simulink model "mc64_hb_43_newquant"  (Simulink 7.6)
settings: Solver=ode45  StartTime=0.0  StopTime=5000  RelTol=1e-3
libraries: xbsIndex_r4 x1281, xps_library x27, casper_library_misc x17, dspsigops x8
(part 1 of 13)
settings Model: Creator=hong  LastModifiedBy=hong

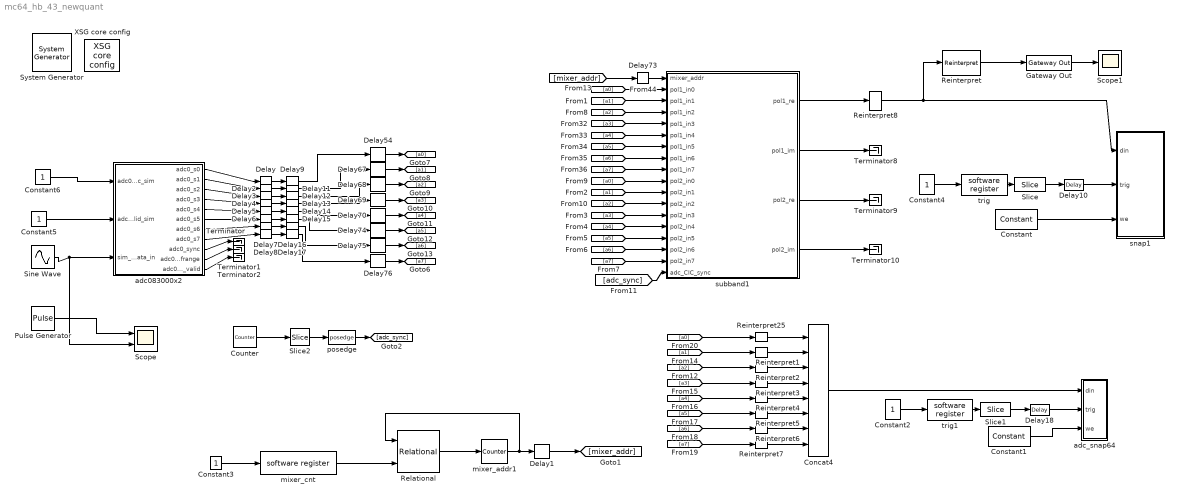
== system mc64_hb_43_newquant ==
  " System Generator" : xbsIndex_r4/ System Generator  Tag=genX  SystemSampleTime=-1  xilinxfamily=virtex5  part=xc5vsx95t  speed=-1  package=ff1136  synthesis_tool=XST  clock_wrapper=Clock Enables  directory=./mc64_hb_43_noise/sysgen  proj_type=Project Navigator  Synth_file=XST Defaults  Impl_file=ISE Defaults  testbench=off  simulink_period=1  sysclk_period=6.6667  dcm_input_clock_period=100  incr_netlist=off  trim_vbits=Everywhere in SubSystem  dbl_ovrd=According to Block Masks  core_generation=According to Block Masks  run_coregen=off  deprecated_control=off  eval_field=0  block_type=sysgen
  Concat4 : xbsIndex_r4/Concat  num_inputs=8  dbl_ovrd=off  block_type=concat
  Constant : xbsIndex_r4/Constant  const=1  gui_display_data_type=Boolean  arith_type=Boolean  n_bits=16  bin_pt=14  preci_type=Single  exp_width=8  frac_width=24  explicit_period=off  period=1  equ=P=C  opselect=C  inp2=PCIN>>17  opr=+  inp1=P  carry=CIN  dbl_ovrd=off  block_type=constant
  Constant1 : xbsIndex_r4/Constant  const=1  gui_display_data_type=Boolean  arith_type=Boolean  n_bits=16  bin_pt=14  preci_type=Single  exp_width=8  frac_width=24  explicit_period=off  period=1  equ=P=C  opselect=C  inp2=PCIN>>17  opr=+  inp1=P  carry=CIN  dbl_ovrd=off  block_type=constant
  Constant{2..6} (5 alike) : Constant
  Counter : xbsIndex_r4/Counter  cnt_type=Free Running  cnt_to=Inf  operation=Up  start_count=0  cnt_by_val=1  arith_type=Unsigned  n_bits=16  bin_pt=0  load_pin=off  rst=off  en=off  explicit_period=on  period=1  dbl_ovrd=off  use_behavioral_HDL=off  implementation=Fabric  block_type=counter
  Delay{,2..8} (8 alike) : xbsIndex_r4/Delay  rst=off  infoeditControl=Selection of Reset will increase slice count due to use of real FFs and instead of SRLs  en=off  latency=3  dbl_ovrd=off  reg_retiming=off  block_type=delay
  Delay1 : xbsIndex_r4/Delay  rst=off  infoeditControl=Selection of Reset will increase slice count due to use of real FFs and instead of SRLs  en=off  latency=2  dbl_ovrd=off  reg_retiming=on  block_type=delay
      settings: block_version=11.4
  Delay10 : xbsIndex_r4/Delay  rst=off  infoeditControl=Selection of Reset will increase slice count due to use of real FFs and instead of SRLs  en=off  latency=20  dbl_ovrd=off  reg_retiming=off  block_type=delay
  Delay{9,11..17} (8 alike) : xbsIndex_r4/Delay  rst=off  infoeditControl=Selection of Reset will increase slice count due to use of real FFs and instead of SRLs  en=off  latency=8  dbl_ovrd=off  reg_retiming=off  block_type=delay
  Delay18 : xbsIndex_r4/Delay  rst=off  infoeditControl=Selection of Reset will increase slice count due to use of real FFs and instead of SRLs  en=off  latency=20  dbl_ovrd=off  reg_retiming=off  block_type=delay
  Delay{54,67..70,74..76} (8 alike) : xbsIndex_r4/Delay  rst=off  infoeditControl=Selection of Reset will increase slice count due to use of real FFs and instead of SRLs  en=off  latency=3  dbl_ovrd=off  reg_retiming=on  block_type=delay
      settings: block_version=11.4
  Delay73 : xbsIndex_r4/Delay  rst=off  infoeditControl=Selection of Reset will increase slice count due to use of real FFs and instead of SRLs  en=off  latency=5  dbl_ovrd=off  reg_retiming=on  block_type=delay
      settings: block_version=11.4
  Gateway Out : xbsIndex_r4/Gateway Out  hdl_port=on  timing_constraint=None  locs_specified=off  LOCs={}  block_type=gatewayout
      settings: infoedit="Gateway out block.  Converts Xilinx fixed point or floating-point type inputs into ouputs of type Simulink integer, double, or fixed point.<br><br>Hardware notes:  In hardware these blocks become top level output ports or are discarded, depending on how they are configured."
  Pulse Generator : DiscretePulseGenerator  Period=480
  Reinterpret : xbsIndex_r4/Reinterpret  force_arith_type=on  arith_type="Signed  (2's comp)"  force_bin_pt=on  bin_pt=31  block_type=reinterpret
  Reinterpret{1..8,25} (9 alike) : xbsIndex_r4/Reinterpret  force_arith_type=on  arith_type=Unsigned  force_bin_pt=on  bin_pt=0  block_type=reinterpret
  Relational : xbsIndex_r4/Relational  mode=a=b  en=off  latency=1  dbl_ovrd=off  block_type=relational
  Scope : Scope  NumInputPorts=2
      settings: YMin=-5~-5  YMax=5~5
  Scope1 : Scope
      settings: TimeRange=746.6442953020135  YMin=-4e-05  YMax=4e-05  SaveName=ScopeData2
  Sine Wave : Sin  Frequency=(pi/2)*(2^1)-(pi/2)*(2^-1)  Samples=200  SampleTime=1/8
  Slice : xbsIndex_r4/Slice  nbits=1  boolean_output=on  mode=Lower Bit Location + Width  bit1=0  base1=MSB of Input  bit0=0  base0=LSB of Input  dbl_ovrd=off  block_type=slice
  Slice1 : xbsIndex_r4/Slice  nbits=1  boolean_output=on  mode=Lower Bit Location + Width  bit1=0  base1=MSB of Input  bit0=0  base0=LSB of Input  dbl_ovrd=off  block_type=slice
  Slice2 : xbsIndex_r4/Slice  nbits=1  boolean_output=on  mode=Upper Bit Location + Width  bit1=0  base1=MSB of Input  bit0=0  base0=LSB of Input  dbl_ovrd=off  block_type=slice
  Terminator{,1..2,8..10} (6 alike) : Terminator
  XSG core config : xps_library/XSG core config  Tag=xps:xsg  SystemSampleTime=-1  hw_sys=ROACH:sx95t  ibob_linux=off  clk_src=adc0_clk  iBOB_clk_src=sys_clk  BEE2_ctrl_clk_src=sys_clk  BEE2_usr_clk_src=sys_clk  ROACH_clk_src=adc0_clk  ROACH2_clk_src=adc0_clk  CORR_clk_src=sys_clk  gpio_clk_io_group=iBOB:sma  gpio_clk_bit_index=0  clk_rate=150  sample_period=1  synthesis_tool=XST  mpc_type=powerpc440_ext
  adc083000x2 : Subsystem  Tag=xps:adc083000x2  AncestorBlock=xps_library/adc083000x2  mask(adc_083000x2){use_adc0=on, use_adc1=off, demux_adc=off, clock_sync=off, verbose=off, using_ctrl=on, adc_clk_rate=800, sample_period=1, bit_width=8}
      mask prompts: use_adc0 "Use ZD0K0?"; use_adc1 "Use ZDOK1?"; demux_adc "Demux ADCs by 2?"; clock_sync "Interleave 2 ADC boards?"; verbose "Verbose Block Creation?"; using_ctrl "Add ports for control registers?"; adc_clk_rate "ADC clock rate (MHz)"; sample_period "Sample Period"; bit_width "Output Bit Width"
      mask help:
      | The ADC block converts analog inputs to digital outputs.
      | Every clock cycle, the inputs are sampled and digitized to
      | 8 bit binary point numbers in the range of [-1, 1).
      |
      | Online block-specific documentation: http://casper.berkeley.edu/wiki/Adc083000
      mask init:
      | adc083000_mask;
      mask Help: eval('xlWeb([getenv(''MLIB_ROOT''), ''\doc\html\sys_adc\sys_adc.html''])')
  adc_snap64 : Subsystem  AncestorBlock=casper_library_scopes/snap64  mask(snap64){nsamples=13}
      mask prompts: nsamples "No. of samples(2^?)"
      mask help:
      | The <i>snap</i> block provides a packaged solution to capturing data from
      | the FPGA fabric and making it accessible from the CPU.  The block comes in
      | 2 flavors: <i>snap</i> (which captures to a 32 bit wide Shared BRAM), and
      | <i>snap64</i> (which captures to 2x32 bit wide Shared BRAMs to effect a
      | 64 bit capture).
      mask Help: eval('xlWeb(''http://casper.berkeley.edu/wiki/Snap'')')
  mixer_addr1 : xbsIndex_r4/Counter  cnt_type=Free Running  cnt_to=Inf  operation=Up  start_count=0  cnt_by_val=1  arith_type=Unsigned  n_bits=11  bin_pt=0  load_pin=off  rst=on  en=off  explicit_period=on  period=1  dbl_ovrd=off  use_behavioral_HDL=off  implementation=Fabric  block_type=counter
      settings: block_version=11.4
  mixer_cnt : xps_library/software register  Tag=xps:sw_reg  SystemSampleTime=-1  io_dir=From Processor  arith_type=Unsigned  bitwidth=32  bin_pt=0  sample_period=1  gw_name=mc64_hb_43_noise_mixer_cnt_user_data_out
  posedge : casper_library_misc/posedge  Tag=Rising Edge Detector  SystemSampleTime=-1
  snap1 : Subsystem  AncestorBlock=casper_library_scopes/snap  mask(snap){nsamples=13}
      mask prompts: nsamples "No. of samples(2^?)"
      mask help:
      | The <i>snap</i> block provides a packaged solution to capturing data from
      | the FPGA fabric and making it accessible from the CPU.  The block comes in
      | 2 flavors: <i>snap</i> (which captures to a 32 bit wide Shared BRAM), and
      | <i>snap64</i> (which captures to 2x32 bit wide Shared BRAMs to effect a
      | 64 bit capture).
      mask Help: eval('xlWeb(''http://casper.berkeley.edu/wiki/Snap'')')
  subband1 : Subsystem  mask{mult_latency=5, add_latency=2, bram_length=10}
      mask prompts: mult_latency "Multiplier Latency"; add_latency "Adder Latency"; bram_length "BRAM Length(2^n)"
  trig : xps_library/software register  Tag=xps:sw_reg  SystemSampleTime=-1  io_dir=From Processor  arith_type=Unsigned  bitwidth=32  bin_pt=0  sample_period=1  gw_name=mc64_hb_43_noise_trig_user_data_out
      link override cic_filter_testing_to_compile_trig_user_data_out: arith_type=Unsigned  n_bits=32  bin_pt=0  period=1
  trig1 : xps_library/software register  Tag=xps:sw_reg  SystemSampleTime=-1  io_dir=From Processor  arith_type=Unsigned  bitwidth=32  bin_pt=0  sample_period=1  gw_name=mc64_hb_43_noise_trig1_user_data_out
      link override cic_filter_testing_to_compile_trig_user_data_out: arith_type=Unsigned  n_bits=32  bin_pt=0  period=1
  wires:
  mixer_addr1/1 -> Delay1/1, Relational/1
  Delay1/1 -> [mixer_addr]
  Relational/1 -> mixer_addr1/1
  mixer_cnt/1 -> Relational/2
  Constant3/1 -> mixer_cnt/1
  [mixer_addr] -> Delay73/1
  [a0] -> subband1/2(pol1_in0)
  [a1] -> subband1/3(pol1_in1)
  [a2] -> subband1/4(pol1_in2)
  [a3] -> subband1/5(pol1_in3)
  [a4] -> subband1/6(pol1_in4)
  [a5] -> subband1/7(pol1_in5)
  [a6] -> subband1/8(pol1_in6)
  [a7] -> subband1/9(pol1_in7)
  [a0] -> subband1/10(pol2_in0)
  [a1] -> subband1/11(pol2_in1)
  [a2] -> subband1/12(pol2_in2)
  [a3] -> subband1/13(pol2_in3)
  [a4] -> subband1/14(pol2_in4)
  [a5] -> subband1/15(pol2_in5)
  [a6] -> subband1/16(pol2_in6)
  [a7] -> subband1/17(pol2_in7)
  Delay73/1 -> subband1/1(mixer_addr)
  subband1/1(pol1_re) -> Reinterpret8/1
  [adc_sync] -> subband1/18(adc_CIC_sync)
  Constant/1 -> snap1/3(we)
  Constant4/1 -> trig/1
  trig/1 -> Slice/1
  Slice/1 -> Delay10/1
  Delay10/1 -> snap1/2(trig)
  Concat4/1 -> adc_snap64/1(din)
  Reinterpret25/1 -> Concat4/1
  Reinterpret1/1 -> Concat4/2
  Reinterpret2/1 -> Concat4/3
  Reinterpret3/1 -> Concat4/4
  Reinterpret4/1 -> Concat4/5
  Reinterpret5/1 -> Concat4/6
  Reinterpret6/1 -> Concat4/7
  Reinterpret7/1 -> Concat4/8
  [a0] -> Reinterpret25/1
  [a1] -> Reinterpret1/1
  [a7] -> Reinterpret7/1
  [a6] -> Reinterpret6/1
  [a5] -> Reinterpret5/1
  [a4] -> Reinterpret4/1
  [a3] -> Reinterpret3/1
  [a2] -> Reinterpret2/1
  Constant1/1 -> adc_snap64/3(we)
  Constant2/1 -> trig1/1
  trig1/1 -> Slice1/1
  Slice1/1 -> Delay18/1
  Delay18/1 -> adc_snap64/2(trig)
  Gateway Out/1 -> Scope1/1
  Reinterpret/1 -> Gateway Out/1
  Reinterpret8/1 -> snap1/1(din), Reinterpret/1
  Sine Wave/1 -> Scope/2, adc083000x2/3(sim_adc0_data_in)
  Pulse Generator/1 -> Scope/1
  adc083000x2/1(adc0_s0) -> Delay/1
  adc083000x2/2(adc0_s1) -> Delay2/1
  adc083000x2/3(adc0_s2) -> Delay3/1
  adc083000x2/4(adc0_s3) -> Delay4/1
  adc083000x2/5(adc0_s4) -> Delay5/1
  adc083000x2/6(adc0_s5) -> Delay6/1
  adc083000x2/7(adc0_s6) -> Delay7/1
  adc083000x2/8(adc0_s7) -> Delay8/1
  Delay54/1 -> [a0]
  Delay67/1 -> [a1]
  Delay68/1 -> [a2]
  Delay69/1 -> [a3]
  Delay70/1 -> [a4]
  Delay74/1 -> [a5]
  Delay75/1 -> [a6]
  Delay76/1 -> [a7]
  Delay/1 -> Delay9/1
  Delay2/1 -> Delay11/1
  Delay3/1 -> Delay12/1
  Delay4/1 -> Delay13/1
  Delay5/1 -> Delay14/1
  Delay6/1 -> Delay15/1
  Delay7/1 -> Delay16/1
  Delay8/1 -> Delay17/1
  Delay9/1 -> Delay54/1
  Delay11/1 -> Delay67/1
  Delay12/1 -> Delay68/1
  Delay13/1 -> Delay69/1
  Delay14/1 -> Delay70/1
  Delay15/1 -> Delay74/1
  Delay16/1 -> Delay75/1
  Delay17/1 -> Delay76/1
  Constant5/1 -> adc083000x2/2(adc0_data_valid_sim)
  adc083000x2/9(adc0_sync) -> Terminator/1
  adc083000x2/10(adc0_outofrange) -> Terminator1/1
  adc083000x2/11(adc0_data_valid) -> Terminator2/1
  Counter/1 -> Slice2/1
  Slice2/1 -> posedge/1
  posedge/1 -> [adc_sync]
  Constant6/1 -> adc083000x2/1(adc0_sync_sim)
  subband1/2(pol1_im) -> Terminator8/1
  subband1/3(pol2_re) -> Terminator9/1
  subband1/4(pol2_im) -> Terminator10/1

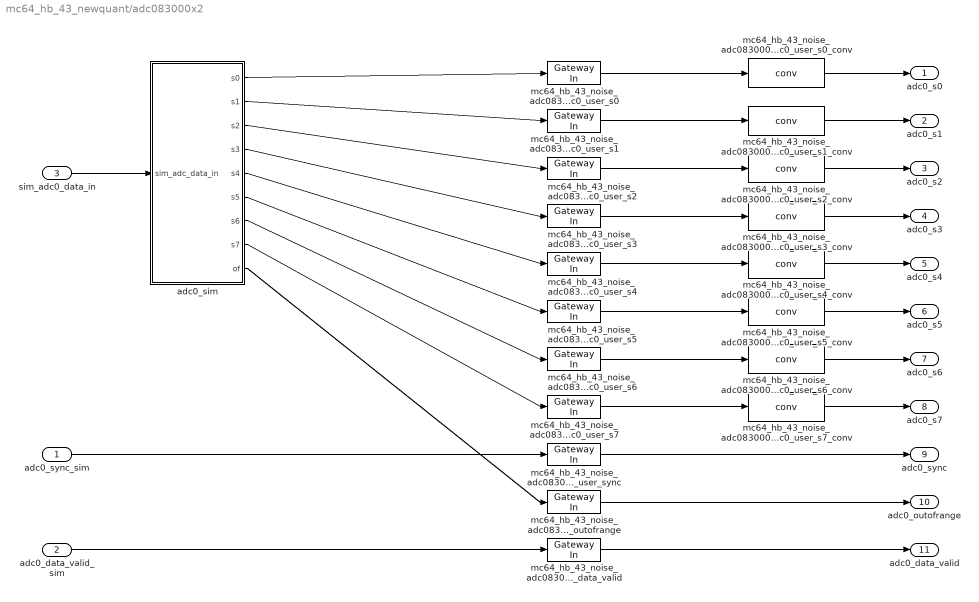
== system mc64_hb_43_newquant/adc083000x2 ==
  adc0_sync_sim : Inport
  adc0_data_valid_sim : Inport  Port=2
  sim_adc0_data_in : Inport  Port=3
  adc0_sim : Subsystem  AncestorBlock=xps_library/ADCs/adc_sim  mask(adc_sim){nStreams=8, bit_width=8}
      mask prompts: nStreams "Number of Output Streams"; bit_width "Sample Bit Width"
      mask help:
      | This block simulates the behavior of a demuxed ADC, which takes
      | as input a waveform and returns digital samples in parallel at
      | a slower rate.
      |
      | This block is used to simulate the behavior
      mask init:
      | adc_sim_init(gcb, ...
      |     'nStreams', nStreams, ...
      |     'bit_width', bit_width);
  mc64_hb_43_noise_adc083000x2_adc0_user_data_valid : xbsIndex_r4/Gateway In  gui_display_data_type=Fixed-point  arith_type=Unsigned  n_bits=1  bin_pt=0  preci_type=Single  exp_width=8  frac_width=24  quantization="Round  (unbiased: +/- Inf)"  overflow=Saturate  period=1  dbl_ovrd=off  timing_constraint=None  locs_specified=off  LOCs={}  hdl_port=on  block_type=gatewayin
      settings: infoedit="Gateway in block.  Converts inputs of type Simulink integer, double and fixed point to  Xilinx fixed point or floating-point data type.<br><br>Hardware notes:  In hardware these blocks become top level input ports."
  mc64_hb_43_noise_adc083000x2_adc0_user_outofrange : xbsIndex_r4/Gateway In  gui_display_data_type=Fixed-point  arith_type=Unsigned  n_bits=4  bin_pt=0  preci_type=Single  exp_width=8  frac_width=24  quantization="Round  (unbiased: +/- Inf)"  overflow=Saturate  period=1  dbl_ovrd=off  timing_constraint=None  locs_specified=off  LOCs={}  hdl_port=on  block_type=gatewayin
      settings: infoedit="Gateway in block.  Converts inputs of type Simulink integer, double and fixed point to  Xilinx fixed point or floating-point data type.<br><br>Hardware notes:  In hardware these blocks become top level input ports."
  mc64_hb_43_noise_adc083000x2_adc0_user_s{0..7} (8 alike) : xbsIndex_r4/Gateway In  gui_display_data_type=Fixed-point  arith_type=Unsigned  n_bits=8  bin_pt=0  preci_type=Single  exp_width=8  frac_width=24  quantization="Round  (unbiased: +/- Inf)"  overflow=Saturate  period=1  dbl_ovrd=off  timing_constraint=None  locs_specified=off  LOCs={}  hdl_port=on  block_type=gatewayin
      settings: infoedit="Gateway in block.  Converts inputs of type Simulink integer, double and fixed point to  Xilinx fixed point or floating-point data type.<br><br>Hardware notes:  In hardware these blocks become top level input ports."
  mc64_hb_43_noise_adc083000x2_adc0_user_s0_conv : xps_library/ADCs/conv  SystemSampleTime=-1  bit_width=8
  mc64_hb_43_noise_adc083000x2_adc0_user_s1_conv : xps_library/ADCs/conv  SystemSampleTime=-1  bit_width=8
  mc64_hb_43_noise_adc083000x2_adc0_user_s2_conv : xps_library/ADCs/conv  SystemSampleTime=-1  bit_width=8
  mc64_hb_43_noise_adc083000x2_adc0_user_s3_conv : xps_library/ADCs/conv  SystemSampleTime=-1  bit_width=8
  mc64_hb_43_noise_adc083000x2_adc0_user_s4_conv : xps_library/ADCs/conv  SystemSampleTime=-1  bit_width=8
  mc64_hb_43_noise_adc083000x2_adc0_user_s5_conv : xps_library/ADCs/conv  SystemSampleTime=-1  bit_width=8
  mc64_hb_43_noise_adc083000x2_adc0_user_s6_conv : xps_library/ADCs/conv  SystemSampleTime=-1  bit_width=8
  mc64_hb_43_noise_adc083000x2_adc0_user_s7_conv : xps_library/ADCs/conv  SystemSampleTime=-1  bit_width=8
  mc64_hb_43_noise_adc083000x2_adc0_user_sync : xbsIndex_r4/Gateway In  gui_display_data_type=Fixed-point  arith_type=Unsigned  n_bits=4  bin_pt=0  preci_type=Single  exp_width=8  frac_width=24  quantization="Round  (unbiased: +/- Inf)"  overflow=Saturate  period=1  dbl_ovrd=off  timing_constraint=None  locs_specified=off  LOCs={}  hdl_port=on  block_type=gatewayin
      settings: infoedit="Gateway in block.  Converts inputs of type Simulink integer, double and fixed point to  Xilinx fixed point or floating-point data type.<br><br>Hardware notes:  In hardware these blocks become top level input ports."
  adc0_s0 : Outport
  adc0_s1 : Outport  Port=2
  adc0_s2 : Outport  Port=3
  adc0_s3 : Outport  Port=4
  adc0_s4 : Outport  Port=5
  adc0_s5 : Outport  Port=6
  adc0_s6 : Outport  Port=7
  adc0_s7 : Outport  Port=8
  adc0_sync : Outport  Port=9
  adc0_outofrange : Outport  Port=10
  adc0_data_valid : Outport  Port=11
  wires:
  sim_adc0_data_in/1 -> adc0_sim/1(sim_adc_data_in)
  adc0_sim/1(s0) -> mc64_hb_43_noise_adc083000x2_adc0_user_s0/1
  mc64_hb_43_noise_adc083000x2_adc0_user_s0/1 -> mc64_hb_43_noise_adc083000x2_adc0_user_s0_conv/1
  mc64_hb_43_noise_adc083000x2_adc0_user_s0_conv/1 -> adc0_s0/1
  adc0_sim/2(s1) -> mc64_hb_43_noise_adc083000x2_adc0_user_s1/1
  mc64_hb_43_noise_adc083000x2_adc0_user_s1/1 -> mc64_hb_43_noise_adc083000x2_adc0_user_s1_conv/1
  mc64_hb_43_noise_adc083000x2_adc0_user_s1_conv/1 -> adc0_s1/1
  adc0_sim/3(s2) -> mc64_hb_43_noise_adc083000x2_adc0_user_s2/1
  mc64_hb_43_noise_adc083000x2_adc0_user_s2/1 -> mc64_hb_43_noise_adc083000x2_adc0_user_s2_conv/1
  mc64_hb_43_noise_adc083000x2_adc0_user_s2_conv/1 -> adc0_s2/1
  adc0_sim/4(s3) -> mc64_hb_43_noise_adc083000x2_adc0_user_s3/1
  mc64_hb_43_noise_adc083000x2_adc0_user_s3/1 -> mc64_hb_43_noise_adc083000x2_adc0_user_s3_conv/1
  mc64_hb_43_noise_adc083000x2_adc0_user_s3_conv/1 -> adc0_s3/1
  adc0_sim/5(s4) -> mc64_hb_43_noise_adc083000x2_adc0_user_s4/1
  mc64_hb_43_noise_adc083000x2_adc0_user_s4/1 -> mc64_hb_43_noise_adc083000x2_adc0_user_s4_conv/1
  mc64_hb_43_noise_adc083000x2_adc0_user_s4_conv/1 -> adc0_s4/1
  adc0_sim/6(s5) -> mc64_hb_43_noise_adc083000x2_adc0_user_s5/1
  mc64_hb_43_noise_adc083000x2_adc0_user_s5/1 -> mc64_hb_43_noise_adc083000x2_adc0_user_s5_conv/1
  mc64_hb_43_noise_adc083000x2_adc0_user_s5_conv/1 -> adc0_s5/1
  adc0_sim/7(s6) -> mc64_hb_43_noise_adc083000x2_adc0_user_s6/1
  mc64_hb_43_noise_adc083000x2_adc0_user_s6/1 -> mc64_hb_43_noise_adc083000x2_adc0_user_s6_conv/1
  mc64_hb_43_noise_adc083000x2_adc0_user_s6_conv/1 -> adc0_s6/1
  adc0_sim/8(s7) -> mc64_hb_43_noise_adc083000x2_adc0_user_s7/1
  mc64_hb_43_noise_adc083000x2_adc0_user_s7/1 -> mc64_hb_43_noise_adc083000x2_adc0_user_s7_conv/1
  mc64_hb_43_noise_adc083000x2_adc0_user_s7_conv/1 -> adc0_s7/1
  adc0_sync_sim/1 -> mc64_hb_43_noise_adc083000x2_adc0_user_sync/1
  mc64_hb_43_noise_adc083000x2_adc0_user_sync/1 -> adc0_sync/1
  adc0_sim/9(of) -> mc64_hb_43_noise_adc083000x2_adc0_user_outofrange/1
  mc64_hb_43_noise_adc083000x2_adc0_user_outofrange/1 -> adc0_outofrange/1
  adc0_data_valid_sim/1 -> mc64_hb_43_noise_adc083000x2_adc0_user_data_valid/1
  mc64_hb_43_noise_adc083000x2_adc0_user_data_valid/1 -> adc0_data_valid/1

== system mc64_hb_43_newquant/adc_snap64 ==
  din : Inport
  trig : Inport  Port=2
  we : Inport  Port=3
  Constant : xbsIndex_r4/Constant  const=1  gui_display_data_type=Fixed-point  arith_type=Boolean  n_bits=1  bin_pt=0  preci_type=Single  exp_width=8  frac_width=24  explicit_period=on  period=1  equ=P=C  opselect=C  inp2=PCIN>>17  opr=+  inp1=P  carry=CIN  dbl_ovrd=off  block_type=constant
      settings: block_version=10.1.1
  Constant1 : xbsIndex_r4/Constant  const=1  gui_display_data_type=Fixed-point  arith_type=Boolean  n_bits=1  bin_pt=0  preci_type=Single  exp_width=8  frac_width=24  explicit_period=on  period=1  equ=P=C  opselect=C  inp2=PCIN>>17  opr=+  inp1=P  carry=CIN  dbl_ovrd=off  block_type=constant
      settings: block_version=10.1.1
  Constant13 : Constant
  Constant2 : xbsIndex_r4/Constant  const=1  gui_display_data_type=Fixed-point  arith_type=Boolean  n_bits=1  bin_pt=0  preci_type=Single  exp_width=8  frac_width=24  explicit_period=on  period=1  equ=P=C  opselect=C  inp2=PCIN>>17  opr=+  inp1=P  carry=CIN  dbl_ovrd=off  block_type=constant
      settings: block_version=10.1.1
  Inverter : xbsIndex_r4/Inverter  en=off  latency=0  dbl_ovrd=off  block_type=inv
      settings: xl_area=[0, 0, 0, 0, 0, 0, 0]  block_version=10.1.1
  Logical1 : xbsIndex_r4/Logical  logical_function=AND  inputs=2  en=off  latency=0  precision=Full  arith_type=Unsigned  n_bits=8  bin_pt=2  align_bp=on  dbl_ovrd=off  block_type=logical
      settings: xl_area=[0, 0, 0, 0, 0, 0, 0]  block_version=10.1.1
  Mux1 : xbsIndex_r4/Mux  inputs=2  en=off  latency=0  precision=Full  arith_type="Signed  (2's comp)"  n_bits=8  bin_pt=2  quantization=Truncate  overflow=Wrap  dbl_ovrd=off  block_type=mux
      settings: xl_area=[0, 0, 0, 0, 0, 0, 0]  block_version=10.1.1
  Mux2 : xbsIndex_r4/Mux  inputs=2  en=off  latency=0  precision=Full  arith_type="Signed  (2's comp)"  n_bits=8  bin_pt=2  quantization=Truncate  overflow=Wrap  dbl_ovrd=off  block_type=mux
      settings: xl_area=[0, 0, 0, 0, 0, 0, 0]  block_version=10.1.1
  Register : xbsIndex_r4/Register  init=0  rst=on  en=on  dbl_ovrd=off  block_type=register
      settings: xl_area=[0, 0, 0, 0, 0, 0, 0]  block_version=10.1.1
  Register1 : xbsIndex_r4/Register  init=0  rst=on  en=on  dbl_ovrd=off  block_type=register
      settings: xl_area=[0, 0, 0, 0, 0, 0, 0]  block_version=10.1.1
  Reinterpret3 : xbsIndex_r4/Reinterpret  force_arith_type=on  arith_type=Unsigned  force_bin_pt=on  bin_pt=0  block_type=reinterpret
      settings: infoedit="Changes signal type without altering the binary representation.   You can changed the signal between signed and unsigned, and relocate the binary point.<P><P>Hardware notes: In hardware this block costs nothing.<P><P>Example:  Suppose the input is 6 bits wide, signed, with 2 fractional bits, and the output is forced to unsigned with 0 fractional bits.  Then an input of -2.0 (1110.00 in binary 2's complement) becomes an output of 56 (111000 in binary)."  block_version=10.1.1
  addr : xps_library/software register  Tag=xps:sw_reg  SystemSampleTime=-1  io_dir=To Processor  arith_type=Unsigned  bitwidth=32  bin_pt=0  sample_period=1  gw_name=mc64_hb_43_noise_adc_snap64_addr_user_data_in
  bram_lsb : Subsystem  Tag=xps:bram  AncestorBlock=xps_library/Shared BRAM  mask{arith_type=Unsigned, addr_width=nsamples, data_width=32, data_bin_pt=0, init_vals=0, sample_rate=1}
      mask prompts: arith_type "Output Data Type"; addr_width "Address width"; data_width "Data Width"; data_bin_pt "Data Binary Point"; init_vals "Initial 32-bit values (simulation only)"; sample_rate "Sample rate"
      mask init:
      | shared_bram_mask;
      mask StyleString: popup(Unsigned|Signed  (2's comp)),edit,popup(8|16|32|64|128),edit,edit,edit
  bram_msb : Subsystem  Tag=xps:bram  AncestorBlock=xps_library/Shared BRAM  mask{arith_type=Unsigned, addr_width=nsamples, data_width=32, data_bin_pt=0, init_vals=0, sample_rate=1}
      mask prompts: arith_type "Output Data Type"; addr_width "Address width"; data_width "Data Width"; data_bin_pt "Data Binary Point"; init_vals "Initial 32-bit values (simulation only)"; sample_rate "Sample rate"
      mask init:
      | shared_bram_mask;
      mask StyleString: popup(Unsigned|Signed  (2's comp)),edit,popup(8|16|32|64|128),edit,edit,edit
  ctrl : xps_library/software register  Tag=xps:sw_reg  SystemSampleTime=-1  io_dir=From Processor  arith_type=Unsigned  bitwidth=32  bin_pt=0  sample_period=1  gw_name=mc64_hb_43_noise_adc_snap64_ctrl_user_data_out
  en1 : xbsIndex_r4/Slice  nbits=32  boolean_output=off  mode=Lower Bit Location + Width  bit1=0  base1=LSB of Input  bit0=32  base0=LSB of Input  dbl_ovrd=off  block_type=slice
      settings: infoedit="Extracts a given range of bits from each input sample and presents it at the output.  The output type is ordinarily unsigned with binary point at zero, but can be Boolean when the slice is one bit wide.<P><P>Hardware notes: In hardware this block costs nothing."  block_version=10.1.1
  en2 : xbsIndex_r4/Slice  nbits=32  boolean_output=off  mode=Lower Bit Location + Width  bit1=0  base1=LSB of Input  bit0=0  base0=LSB of Input  dbl_ovrd=off  block_type=slice
      settings: infoedit="Extracts a given range of bits from each input sample and presents it at the output.  The output type is ordinarily unsigned with binary point at zero, but can be Boolean when the slice is one bit wide.<P><P>Hardware notes: In hardware this block costs nothing."  block_version=10.1.1
  enable : xbsIndex_r4/Slice  nbits=1  boolean_output=on  mode=Lower Bit Location + Width  bit1=0  base1=LSB of Input  bit0=0  base0=LSB of Input  dbl_ovrd=off  block_type=slice
      settings: infoedit="Extracts a given range of bits from each input sample and presents it at the output.  The output type is ordinarily unsigned with binary point at zero, but can be Boolean when the slice is one bit wide.<P><P>Hardware notes: In hardware this block costs nothing."  block_version=10.1.1
  freeze_cntr : casper_library_misc/freeze_cntr  SystemSampleTime=-1  CounterBits=nsamples
  posedge : casper_library_misc/posedge  Tag=Rising Edge Detector  SystemSampleTime=-1
  trig1 : xbsIndex_r4/Slice  nbits=1  boolean_output=on  mode=Lower Bit Location + Width  bit1=0  base1=LSB of Input  bit0=1  base0=LSB of Input  dbl_ovrd=off  block_type=slice
      settings: infoedit="Extracts a given range of bits from each input sample and presents it at the output.  The output type is ordinarily unsigned with binary point at zero, but can be Boolean when the slice is one bit wide.<P><P>Hardware notes: In hardware this block costs nothing."  block_version=10.1.1
  valid : xbsIndex_r4/Slice  nbits=1  boolean_output=on  mode=Lower Bit Location + Width  bit1=0  base1=LSB of Input  bit0=2  base0=LSB of Input  dbl_ovrd=off  block_type=slice
      settings: infoedit="Extracts a given range of bits from each input sample and presents it at the output.  The output type is ordinarily unsigned with binary point at zero, but can be Boolean when the slice is one bit wide.<P><P>Hardware notes: In hardware this block costs nothing."  block_version=10.1.1
  wires:
  en2/1 -> bram_lsb/2(data_in)
  en1/1 -> bram_msb/2(data_in)
  din/1 -> Reinterpret3/1
  Reinterpret3/1 -> en2/1, en1/1
  trig/1 -> Mux2/2
  enable/1 -> posedge/1
  freeze_cntr/2 -> Register1/3, bram_msb/3(we), bram_lsb/3(we)
  Constant13/1 -> ctrl/1
  ctrl/1 -> enable/1, valid/1, trig1/1
  posedge/1 -> Register/3, Register1/2, Inverter/1
  Constant/1 -> Register/1
  Constant1/1 -> Mux2/3
  Mux1/1 -> freeze_cntr/1
  we/1 -> Mux1/2
  Constant2/1 -> Mux1/3
  Register1/1 -> addr/1
  trig1/1 -> Mux2/1
  valid/1 -> Mux1/1
  Logical1/1 -> Register/2
  Inverter/1 -> Logical1/2
  Mux2/1 -> Logical1/1
  Register/1 -> freeze_cntr/2
  freeze_cntr/1 -> Register1/1, bram_msb/1(addr), bram_lsb/1(addr)

== system mc64_hb_43_newquant/snap1 ==
  din : Inport
  trig : Inport  Port=2
  we : Inport  Port=3
  Constant : xbsIndex_r4/Constant  const=1  gui_display_data_type=Fixed-point  arith_type=Boolean  n_bits=1  bin_pt=0  preci_type=Single  exp_width=8  frac_width=24  explicit_period=on  period=1  equ=P=C  opselect=C  inp2=PCIN>>17  opr=+  inp1=P  carry=CIN  dbl_ovrd=off  block_type=constant
      settings: block_version=10.1.1
  Constant1 : xbsIndex_r4/Constant  const=1  gui_display_data_type=Fixed-point  arith_type=Boolean  n_bits=1  bin_pt=0  preci_type=Single  exp_width=8  frac_width=24  explicit_period=on  period=1  equ=P=C  opselect=C  inp2=PCIN>>17  opr=+  inp1=P  carry=CIN  dbl_ovrd=off  block_type=constant
      settings: block_version=10.1.1
  Constant13 : Constant
  Constant2 : xbsIndex_r4/Constant  const=1  gui_display_data_type=Fixed-point  arith_type=Boolean  n_bits=1  bin_pt=0  preci_type=Single  exp_width=8  frac_width=24  explicit_period=on  period=1  equ=P=C  opselect=C  inp2=PCIN>>17  opr=+  inp1=P  carry=CIN  dbl_ovrd=off  block_type=constant
      settings: block_version=10.1.1
  Inverter : xbsIndex_r4/Inverter  en=off  latency=0  dbl_ovrd=off  block_type=inv
      settings: xl_area=[0, 0, 0, 0, 0, 0, 0]  block_version=10.1.1
  Logical1 : xbsIndex_r4/Logical  logical_function=AND  inputs=2  en=off  latency=0  precision=Full  arith_type=Unsigned  n_bits=8  bin_pt=2  align_bp=on  dbl_ovrd=off  block_type=logical
      settings: xl_area=[0, 0, 0, 0, 0, 0, 0]  block_version=10.1.1
  Mux1 : xbsIndex_r4/Mux  inputs=2  en=off  latency=0  precision=Full  arith_type="Signed  (2's comp)"  n_bits=8  bin_pt=2  quantization=Truncate  overflow=Wrap  dbl_ovrd=off  block_type=mux
      settings: xl_area=[0, 0, 0, 0, 0, 0, 0]  block_version=10.1.1
  Mux2 : xbsIndex_r4/Mux  inputs=2  en=off  latency=0  precision=Full  arith_type="Signed  (2's comp)"  n_bits=8  bin_pt=2  quantization=Truncate  overflow=Wrap  dbl_ovrd=off  block_type=mux
      settings: xl_area=[0, 0, 0, 0, 0, 0, 0]  block_version=10.1.1
  Register : xbsIndex_r4/Register  init=0  rst=on  en=on  dbl_ovrd=off  block_type=register
      settings: xl_area=[0, 0, 0, 0, 0, 0, 0]  block_version=10.1.1
  Register1 : xbsIndex_r4/Register  init=0  rst=on  en=on  dbl_ovrd=off  block_type=register
      settings: xl_area=[0, 0, 0, 0, 0, 0, 0]  block_version=10.1.1
  Reinterpret : xbsIndex_r4/Reinterpret  force_arith_type=on  arith_type=Unsigned  force_bin_pt=on  bin_pt=0  block_type=reinterpret
      settings: infoedit="Changes signal type without altering the binary representation.   You can changed the signal between signed and unsigned, and relocate the binary point.<P><P>Hardware notes: In hardware this block costs nothing.<P><P>Example:  Suppose the input is 6 bits wide, signed, with 2 fractional bits, and the output is forced to unsigned with 0 fractional bits.  Then an input of -2.0 (1110.00 in binary 2's complement) becomes an output of 56 (111000 in binary)."  block_version=10.1.1
  addr : xps_library/software register  Tag=xps:sw_reg  SystemSampleTime=-1  io_dir=To Processor  arith_type=Unsigned  bitwidth=32  bin_pt=0  sample_period=1  gw_name=mc64_hb_43_noise_snap1_addr_user_data_in
  bram : Subsystem  Tag=xps:bram  AncestorBlock=xps_library/Shared BRAM  mask{arith_type=Unsigned, addr_width=nsamples, data_width=32, data_bin_pt=0, init_vals=0, sample_rate=1}
      mask prompts: arith_type "Output Data Type"; addr_width "Address width"; data_width "Data Width"; data_bin_pt "Data Binary Point"; init_vals "Initial 32-bit values (simulation only)"; sample_rate "Sample rate"
      mask init:
      | shared_bram_mask;
      mask StyleString: popup(Unsigned|Signed  (2's comp)),edit,popup(8|16|32|64|128),edit,edit,edit
  ctrl : xps_library/software register  Tag=xps:sw_reg  SystemSampleTime=-1  io_dir=From Processor  arith_type=Unsigned  bitwidth=32  bin_pt=0  sample_period=1  gw_name=mc64_hb_43_noise_snap1_ctrl_user_data_out
  enable : xbsIndex_r4/Slice  nbits=1  boolean_output=on  mode=Lower Bit Location + Width  bit1=0  base1=LSB of Input  bit0=0  base0=LSB of Input  dbl_ovrd=off  block_type=slice
      settings: infoedit="Extracts a given range of bits from each input sample and presents it at the output.  The output type is ordinarily unsigned with binary point at zero, but can be Boolean when the slice is one bit wide.<P><P>Hardware notes: In hardware this block costs nothing."  block_version=10.1.1
  freeze_cntr : casper_library_misc/freeze_cntr  SystemSampleTime=-1  CounterBits=nsamples
  posedge : casper_library_misc/posedge  Tag=Rising Edge Detector  SystemSampleTime=-1
  trig1 : xbsIndex_r4/Slice  nbits=1  boolean_output=on  mode=Lower Bit Location + Width  bit1=0  base1=LSB of Input  bit0=1  base0=LSB of Input  dbl_ovrd=off  block_type=slice
      settings: infoedit="Extracts a given range of bits from each input sample and presents it at the output.  The output type is ordinarily unsigned with binary point at zero, but can be Boolean when the slice is one bit wide.<P><P>Hardware notes: In hardware this block costs nothing."  block_version=10.1.1
  valid : xbsIndex_r4/Slice  nbits=1  boolean_output=on  mode=Lower Bit Location + Width  bit1=0  base1=LSB of Input  bit0=2  base0=LSB of Input  dbl_ovrd=off  block_type=slice
      settings: infoedit="Extracts a given range of bits from each input sample and presents it at the output.  The output type is ordinarily unsigned with binary point at zero, but can be Boolean when the slice is one bit wide.<P><P>Hardware notes: In hardware this block costs nothing."  block_version=10.1.1
  wires:
  trig/1 -> Mux2/2
  freeze_cntr/1 -> Register1/1, bram/1(addr)
  enable/1 -> posedge/1
  Register/1 -> freeze_cntr/2
  freeze_cntr/2 -> bram/3(we), Register1/3
  Constant13/1 -> ctrl/1
  Reinterpret/1 -> bram/2(data_in)
  din/1 -> Reinterpret/1
  ctrl/1 -> enable/1, valid/1, trig1/1
  posedge/1 -> Register/3, Register1/2, Inverter/1
  Constant/1 -> Register/1
  Constant1/1 -> Mux2/3
  Mux1/1 -> freeze_cntr/1
  we/1 -> Mux1/2
  Constant2/1 -> Mux1/3
  Register1/1 -> addr/1
  trig1/1 -> Mux2/1
  valid/1 -> Mux1/1
  Logical1/1 -> Register/2
  Inverter/1 -> Logical1/2
  Mux2/1 -> Logical1/1
